simulink model "broadwayIPC_2024b"  (R2024b)
settings: Solver=FixedStepDiscrete  StartTime=0.0  StopTime=2  RelTol=1e-3
undefined symbols (not defined in the file or in its folder): gray
libraries: hdlsllib x26, visionhdlio x6, visionsources x2
Description:
  | Sobel Edge Detection Using the MATLAB(R) Function Block
  | This example shows how to use HDL Coder(TM) to check,
  | generate, and verify HDL code for a Sobel Edge Detection
  | block built using the MATLAB Function block.
settings Model: Creator=The MathWorks, Inc.  LastModifiedBy=Chris
settings SolverCC: AlgebraicLoopSolver=TrustRegion
settings DataIOCC: LimitDataPoints=on  SaveFormat=Array  SignalLogging=off  ReturnWorkspaceOutputs=off
settings OptimizationCC: BlockReduction=off  ConditionallyExecuteInputs=off  DefaultParameterBehavior=Inlined  ExpressionDepthLimit=2147483647  InitFltsAndDblsToZero=on  EfficientMapNaN2IntZero=off  LifeSpan=inf
settings DebuggingCC: AlgebraicLoopMsg=error  SaveWithParameterizedLinksMsg=none  UnderspecifiedInitializationDetection=Classic  MergeDetectMultiDrivingBlocksExec=none  SignalResolutionControl=TryResolveAllWithWarning  MultiTaskDSMMsg=warning  MultiTaskCondExecSysMsg=none  SingleTaskRateTransMsg=error  IntegerOverflowMsg=none  ParameterPrecisionLossMsg=none  FcnCallInpInsideContextMsg=warning  UnconnectedInputMsg=warning  UnconnectedOutputMsg=warning  UnconnectedLineMsg=warning  AllowSymbolicDim=off  StateNameClashWarn=warning  StrictBusMsg=ErrorOnBusTreatedAsVector  SFUnexpectedBacktrackingDiag=warning  SFNoUnconditionalDefaultTransitionDiag=warning  SFExecutionAtInitializationDiag=none  IntegerSaturationMsg=none  ArithmeticOperatorsInVariantConditions=warning
settings HardwareCC: ProdBitPerPointer=32  ProdBitPerSizeT=32  ProdBitPerPtrDiffT=32  ProdLargestAtomicFloat=None  ProdIntDivRoundTo=Undefined  ProdEndianess=Unspecified  ProdWordSize=32  ProdHWDeviceType=ASIC/FPGA  TargetHWDeviceType=32-bit Generic  ProdEqTarget=off
settings ModelReferenceCC: EnableRefExpFcnMdlSchedulingChecks=on  PropagateSignalLabelsOutOfModel=off
settings SFSimCC: SimUseLocalCustomCode=off  CustomCodeUndefinedFunction=UseInterfaceOnly
settings RTWCC: RTWUseLocalCustomCode=off  GPUComputeCapability=3.5  DLArmComputeVersion=19.05
settings CodeAppCC: StateflowObjectComments=on
settings GRTTargetCC: TargetFcnLib=ansi_tfl_tmw.mat  TargetLangStandard=C89/C90 (ANSI)  CombineOutputUpdateFcns=off  GRTInterface=on
settings ConfigComp: CovMetricSettings=dw  CovSaveCumulativeToWorkspaceVar=on  CovSaveSingleToWorkspaceVar=on  CovExternalEMLEnable=off

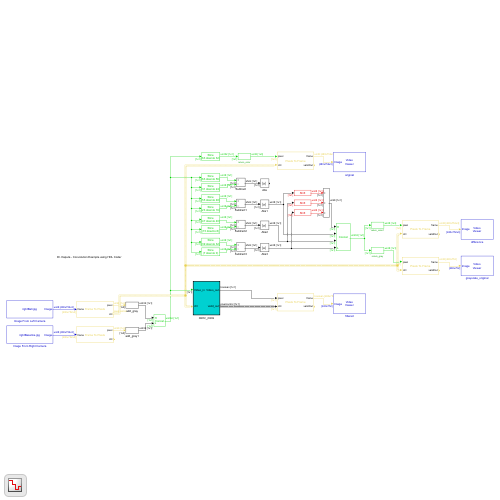
[thumbnail: Simulink's stored preview of the top-level diagram]
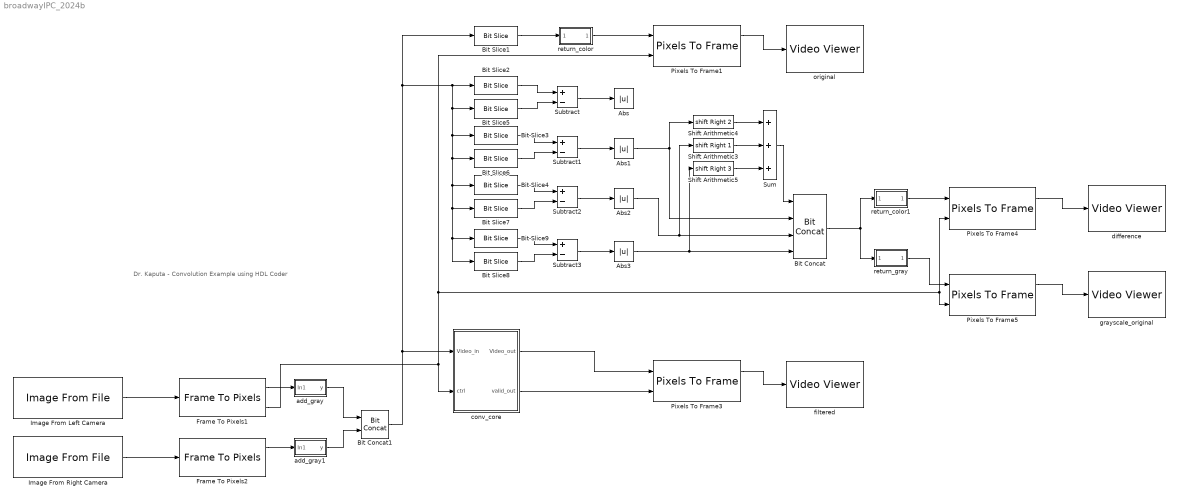
== system broadwayIPC_2024b ==
  note: Dr. Kaputa - Convolution Example using HDL Coder
  Abs{,1..3} (4 alike) : Abs  OutDataTypeStr=uint8
  Bit Concat : hdlsllib/Logic and Bit Operations/Bit Concat  numInputs=4
  Bit Concat1 : hdlsllib/Logic and Bit Operations/Bit Concat  numInputs=2
  Bit Slice1 : hdlsllib/Logic and Bit Operations/Bit Slice  lidx=63  ridx=32
  Bit Slice2 : hdlsllib/Logic and Bit Operations/Bit Slice  lidx=63  ridx=56
  Bit Slice3 : hdlsllib/Logic and Bit Operations/Bit Slice  lidx=55  ridx=48
  Bit Slice4 : hdlsllib/Logic and Bit Operations/Bit Slice  lidx=47  ridx=40
  Bit Slice5 : hdlsllib/Logic and Bit Operations/Bit Slice  lidx=31  ridx=24
  Bit Slice6 : hdlsllib/Logic and Bit Operations/Bit Slice  lidx=23  ridx=16
  Bit Slice7 : hdlsllib/Logic and Bit Operations/Bit Slice  lidx=15  ridx=8
  Bit Slice8 : hdlsllib/Logic and Bit Operations/Bit Slice  lidx=7  ridx=0
  Bit Slice9 : hdlsllib/Logic and Bit Operations/Bit Slice  lidx=39  ridx=32
  Frame To Pixels1 : visionhdlio/Frame To Pixels  NumComponents=3  NumPixels=1  VideoFormat=Custom  ActivePixelsPerLine=R  ActiveVideoLines=C  TotalPixelsPerLine=R  TotalVideoLines=C  StartingActiveLine=1  FrontPorch=0  SampleTime=0  VideoFormatCache=Custom  ActivePixelsPerLineCache=R  ActiveVideoLinesCache=C  TotalPixelsPerLineCache=R  TotalVideoLinesCache=C  StartingActiveLineCache=1  FrontPorchCache=0
  Frame To Pixels2 : visionhdlio/Frame To Pixels  NumComponents=3  NumPixels=1  VideoFormat=Custom  ActivePixelsPerLine=R  ActiveVideoLines=C  TotalPixelsPerLine=R  TotalVideoLines=C  StartingActiveLine=1  FrontPorch=0  SampleTime=0  VideoFormatCache=Custom  ActivePixelsPerLineCache=R  ActiveVideoLinesCache=C  TotalPixelsPerLineCache=R  TotalVideoLinesCache=C  StartingActiveLineCache=1  FrontPorchCache=0
  Image From Left Camera : visionsources/Image From File  Tag=vipblks_nd  FileName=C:\Users\Chris\Documents\Repos\WiiSports\TennisTracker\BoradwaySimulink\rightBall.jpg  Ts=1  imagePorts=One multidimensional signal  OutPortLabels=R|G|B  ImageDataType=Inherit from input image  sdImageDataType=uint(8)  Signed=on  WordLength=16  FractionLengthMode=User-defined  FractionLength=15
  Image From Right Camera : visionsources/Image From File  Tag=vipblks_nd  FileName=C:\Users\Chris\Documents\Repos\WiiSports\TennisTracker\BoradwaySimulink\rightBaseline.jpg  Ts=1  imagePorts=One multidimensional signal  OutPortLabels=R|G|B  ImageDataType=Inherit from input image  sdImageDataType=uint(8)  Signed=on  WordLength=16  FractionLengthMode=User-defined  FractionLength=15
  Pixels To Frame1 : visionhdlio/Pixels To Frame  NumComponents=3  NumPixels=1  VideoFormat=Custom  ActivePixelsPerLine=R  ActiveVideoLines=C  TotalPixelsPerLine=R  TotalVideoLines=C  VideoFormatCache=Custom  ActivePixelsPerLineCache=R  ActiveVideoLinesCache=C  TotalPixelsPerLineCache=R  TotalVideoLinesCache=C
  Pixels To Frame3 : visionhdlio/Pixels To Frame  NumComponents=1  NumPixels=1  VideoFormat=Custom  ActivePixelsPerLine=R  ActiveVideoLines=C  TotalPixelsPerLine=R  TotalVideoLines=C  VideoFormatCache=Custom  ActivePixelsPerLineCache=R  ActiveVideoLinesCache=C  TotalPixelsPerLineCache=R  TotalVideoLinesCache=C
  Pixels To Frame4 : visionhdlio/Pixels To Frame  NumComponents=3  NumPixels=1  VideoFormat=Custom  ActivePixelsPerLine=R  ActiveVideoLines=C  TotalPixelsPerLine=R  TotalVideoLines=C  VideoFormatCache=Custom  ActivePixelsPerLineCache=R  ActiveVideoLinesCache=C  TotalPixelsPerLineCache=R  TotalVideoLinesCache=C
  Pixels To Frame5 : visionhdlio/Pixels To Frame  NumComponents=1  NumPixels=1  VideoFormat=Custom  ActivePixelsPerLine=R  ActiveVideoLines=C  TotalPixelsPerLine=R  TotalVideoLines=C  VideoFormatCache=Custom  ActivePixelsPerLineCache=R  ActiveVideoLinesCache=C  TotalPixelsPerLineCache=R  TotalVideoLinesCache=C
  Shift Arithmetic3 : ArithShift  BitShiftNumber=1  BitShiftDirection=Right
  Shift Arithmetic4 : ArithShift  BitShiftNumber=2  BitShiftDirection=Right
  Shift Arithmetic5 : ArithShift  BitShiftNumber=3  BitShiftDirection=Right
  Subtract{,1..3} (4 alike) : Sum  Inputs=+-
  Sum : Sum  Inputs=+++  OutDataTypeStr=uint8
  add_gray : Subsystem
  add_gray1 : Subsystem
  conv_core : Subsystem  TreatAsAtomicUnit=on
  difference : VideoViewer  FigPos=[994 1078 927 429]
  filtered : VideoViewer  colormapValue=gray(256)  FigPos=[66 1078 927 429]
  grayscale_original : VideoViewer  FigPos=[65 538 927 429]
  original : VideoViewer  FigPos=[995 538 927 429]
  return_color : Subsystem
  return_color1 : Subsystem
  return_gray : Subsystem
  wires:
  Image From Left Camera/1 -> Frame To Pixels1/1
  Pixels To Frame1/1 -> original/1
  return_color/1(RGBVector) -> Pixels To Frame1/1
  Frame To Pixels1/1 -> add_gray/1(In1)
  Pixels To Frame3/1 -> filtered/1
  conv_core/2(valid_out) -> Pixels To Frame3/2
  Bit Concat1/1 -> Bit Slice1/1, Bit Slice2/1, Bit Slice8/1, Bit Slice9/1, Bit Slice7/1, Bit Slice4/1, Bit Slice6/1, Bit Slice3/1, Bit Slice5/1, conv_core/1(Video_in)
  conv_core/1(Video_out) -> Pixels To Frame3/1
  Image From Right Camera/1 -> Frame To Pixels2/1
  Frame To Pixels1/2 -> Pixels To Frame1/2, Pixels To Frame5/2, Pixels To Frame4/2, conv_core/2(ctrl)
  Frame To Pixels2/1 -> add_gray1/1(In1)
  add_gray/1(y) -> Bit Concat1/1
  add_gray1/1(y) -> Bit Concat1/2
  Bit Slice1/1 -> return_color/1(RGB)
  Pixels To Frame4/1 -> difference/1
  Subtract/1 -> Abs/1
  return_color1/1(RGBVector) -> Pixels To Frame4/1
  Subtract1/1 -> Abs1/1
  Subtract2/1 -> Abs2/1
  Subtract3/1 -> Abs3/1
  Bit Slice2/1 -> Subtract/1
  Bit Slice5/1 -> Subtract/2
  Bit Slice3/1 -> Subtract1/1
  Bit Slice6/1 -> Subtract1/2
  Bit Slice4/1 -> Subtract2/1
  Bit Slice7/1 -> Subtract2/2
  Bit Slice9/1 -> Subtract3/1
  Bit Slice8/1 -> Subtract3/2
  Pixels To Frame5/1 -> grayscale_original/1
  return_gray/1(RGBVector) -> Pixels To Frame5/1
  Shift Arithmetic5/1 -> Sum/3
  Shift Arithmetic3/1 -> Sum/2
  Shift Arithmetic4/1 -> Sum/1
  Abs3/1 -> Shift Arithmetic5/1, Bit Concat/4
  Abs2/1 -> Shift Arithmetic3/1, Bit Concat/3
  Abs1/1 -> Shift Arithmetic4/1, Bit Concat/2
  Sum/1 -> Bit Concat/1
  Bit Concat/1 -> return_gray/1(RGB), return_color1/1(RGB)

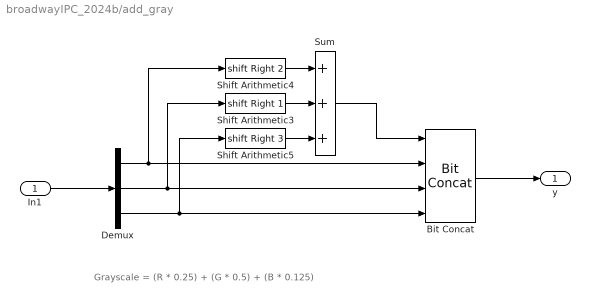
== system broadwayIPC_2024b/add_gray ==
  note: Grayscale = (R * 0.25) + (G * 0.5) + (B * 0.125)
  In1 : Inport
  Bit Concat : hdlsllib/Logic and Bit Operations/Bit Concat  numInputs=4
  Demux : Demux  Outputs=3
  Shift Arithmetic3 : ArithShift  BitShiftNumber=1  BitShiftDirection=Right
  Shift Arithmetic4 : ArithShift  BitShiftNumber=2  BitShiftDirection=Right
  Shift Arithmetic5 : ArithShift  BitShiftNumber=3  BitShiftDirection=Right
  Sum : Sum  Inputs=+++  OutDataTypeStr=uint8
  y : Outport
  wires:
  Bit Concat/1 -> y/1
  In1/1 -> Demux/1
  Demux/2 -> Shift Arithmetic3/1, Bit Concat/3
  Demux/1 -> Shift Arithmetic4/1, Bit Concat/2
  Demux/3 -> Shift Arithmetic5/1, Bit Concat/4
  Sum/1 -> Bit Concat/1
  Shift Arithmetic4/1 -> Sum/1
  Shift Arithmetic3/1 -> Sum/2
  Shift Arithmetic5/1 -> Sum/3

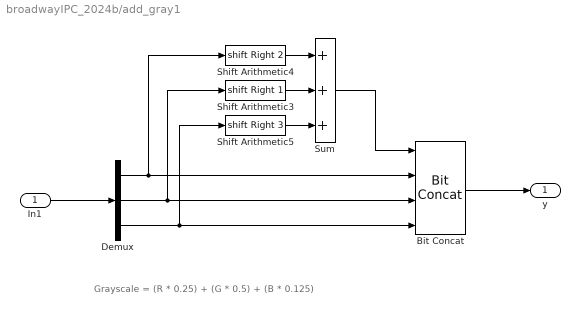
== system broadwayIPC_2024b/add_gray1 ==
  note: Grayscale = (R * 0.25) + (G * 0.5) + (B * 0.125)
  In1 : Inport
  Bit Concat : hdlsllib/Logic and Bit Operations/Bit Concat  numInputs=4
  Demux : Demux  Outputs=3
  Shift Arithmetic3 : ArithShift  BitShiftNumber=1  BitShiftDirection=Right
  Shift Arithmetic4 : ArithShift  BitShiftNumber=2  BitShiftDirection=Right
  Shift Arithmetic5 : ArithShift  BitShiftNumber=3  BitShiftDirection=Right
  Sum : Sum  Inputs=+++  OutDataTypeStr=uint8
  y : Outport
  wires:
  Bit Concat/1 -> y/1
  In1/1 -> Demux/1
  Demux/2 -> Shift Arithmetic3/1, Bit Concat/3
  Demux/1 -> Shift Arithmetic4/1, Bit Concat/2
  Demux/3 -> Shift Arithmetic5/1, Bit Concat/4
  Shift Arithmetic4/1 -> Sum/1
  Shift Arithmetic3/1 -> Sum/2
  Shift Arithmetic5/1 -> Sum/3
  Sum/1 -> Bit Concat/1

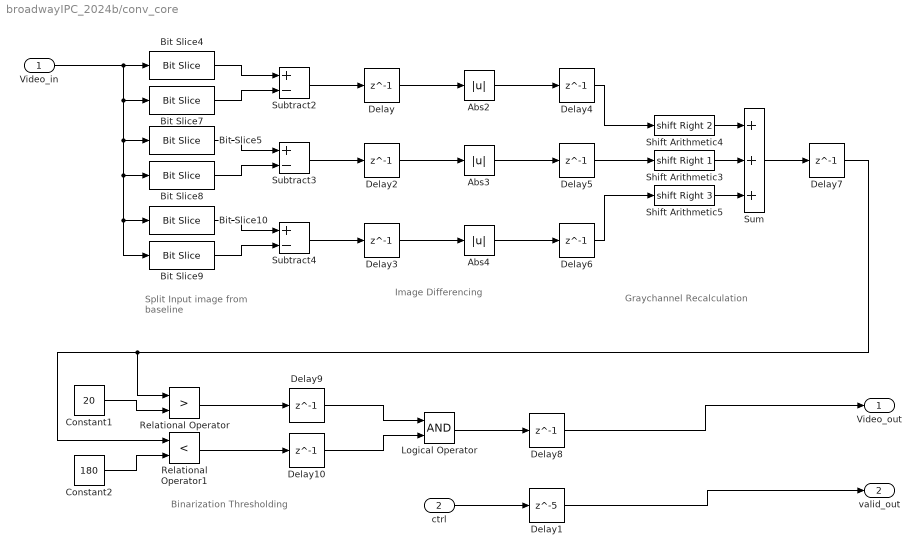
== system broadwayIPC_2024b/conv_core ==
  note: Graychannel Recalculation
  note: Split Input image
      | from baseline
  note: Image
      | Differencing
  note: Binarization Thresholding
  Video_in : Inport
  ctrl : Inport  Port=2
  Abs2 : Abs  OutDataTypeStr=uint8  SaturateOnIntegerOverflow=off
  Abs3 : Abs  OutDataTypeStr=uint8  SaturateOnIntegerOverflow=off
  Abs4 : Abs  OutDataTypeStr=uint8  SaturateOnIntegerOverflow=off
  Bit Slice10 : hdlsllib/Logic and Bit Operations/Bit Slice  lidx=39  ridx=32
  Bit Slice4 : hdlsllib/Logic and Bit Operations/Bit Slice  lidx=55  ridx=48
  Bit Slice5 : hdlsllib/Logic and Bit Operations/Bit Slice  lidx=47  ridx=40
  Bit Slice7 : hdlsllib/Logic and Bit Operations/Bit Slice  lidx=23  ridx=16
  Bit Slice8 : hdlsllib/Logic and Bit Operations/Bit Slice  lidx=15  ridx=8
  Bit Slice9 : hdlsllib/Logic and Bit Operations/Bit Slice  lidx=7  ridx=0
  Constant1 : Constant  Value=20  OutDataTypeStr=uint8
  Constant2 : Constant  Value=180  OutDataTypeStr=uint8
  Delay{,2..10} (10 alike) : Delay  DelayLength=1  InitialCondition=0
  Delay1 : Delay  DelayLength=5  InitialCondition=0
  Logical Operator : Logic  AllPortsSameDT=off  OutDataTypeStr=boolean
  Relational Operator : RelationalOperator  Operator=>  OutDataTypeStr=boolean  RndMeth=Simplest  InputSameDT=off
  Relational Operator1 : RelationalOperator  Operator=<  OutDataTypeStr=boolean  RndMeth=Simplest  InputSameDT=off
  Shift Arithmetic3 : ArithShift  BitShiftNumber=1  BitShiftDirection=Right
  Shift Arithmetic4 : ArithShift  BitShiftNumber=2  BitShiftDirection=Right
  Shift Arithmetic5 : ArithShift  BitShiftNumber=3  BitShiftDirection=Right
  Subtract2 : Sum  Inputs=+-
  Subtract3 : Sum  Inputs=+-
  Subtract4 : Sum  Inputs=+-
  Sum : Sum  Inputs=+++  OutDataTypeStr=uint8
  Video_out : Outport  VectorParamsAs1DForOutWhenUnconnected=off
  valid_out : Outport  Port=2  VectorParamsAs1DForOutWhenUnconnected=off
  wires:
  ctrl/1 -> Delay1/1
  Constant1/1 -> Relational Operator/2
  Constant2/1 -> Relational Operator1/2
  Abs2/1 -> Delay4/1
  Bit Slice9/1 -> Subtract4/2
  Bit Slice7/1 -> Subtract2/2
  Bit Slice4/1 -> Subtract2/1
  Bit Slice10/1 -> Subtract4/1
  Abs3/1 -> Delay5/1
  Bit Slice5/1 -> Subtract3/1
  Bit Slice8/1 -> Subtract3/2
  Abs4/1 -> Delay6/1
  Video_in/1 -> Bit Slice9/1, Bit Slice10/1, Bit Slice8/1, Bit Slice5/1, Bit Slice7/1, Bit Slice4/1
  Sum/1 -> Delay7/1
  Shift Arithmetic4/1 -> Sum/1
  Shift Arithmetic5/1 -> Sum/3
  Shift Arithmetic3/1 -> Sum/2
  Subtract2/1 -> Delay/1
  Delay/1 -> Abs2/1
  Subtract3/1 -> Delay2/1
  Delay2/1 -> Abs3/1
  Subtract4/1 -> Delay3/1
  Delay3/1 -> Abs4/1
  Delay4/1 -> Shift Arithmetic4/1
  Delay5/1 -> Shift Arithmetic3/1
  Delay6/1 -> Shift Arithmetic5/1
  Delay7/1 -> Relational Operator/1, Relational Operator1/1
  Logical Operator/1 -> Delay8/1
  Relational Operator/1 -> Delay9/1
  Relational Operator1/1 -> Delay10/1
  Delay10/1 -> Logical Operator/2
  Delay9/1 -> Logical Operator/1
  Delay8/1 -> Video_out/1
  Delay1/1 -> valid_out/1

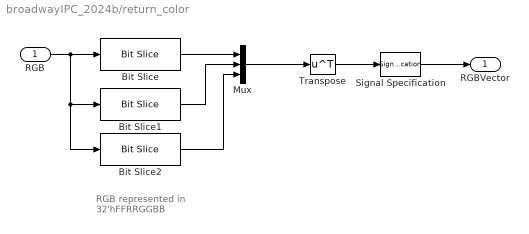
== system broadwayIPC_2024b/return_color ==
  note: RGB represented in
      | 32'hFFRRGGBB
  RGB : Inport
  Bit Slice : hdlsllib/Logic and Bit Operations/Bit Slice  lidx=23  ridx=16
  Bit Slice1 : hdlsllib/Logic and Bit Operations/Bit Slice  lidx=15  ridx=8
  Bit Slice2 : hdlsllib/Logic and Bit Operations/Bit Slice  lidx=7  ridx=0
  Mux : Mux  Inputs=3
  Signal Specification : SignalSpecification
  Transpose : Math  Operator=transpose  SignedPower=on
  RGBVector : Outport  VectorParamsAs1DForOutWhenUnconnected=off
  wires:
  Signal Specification/1 -> RGBVector/1
  Transpose/1 -> Signal Specification/1
  RGB/1 -> Bit Slice/1, Bit Slice1/1, Bit Slice2/1
  Bit Slice1/1 -> Mux/2
  Bit Slice2/1 -> Mux/3
  Bit Slice/1 -> Mux/1
  Mux/1 -> Transpose/1

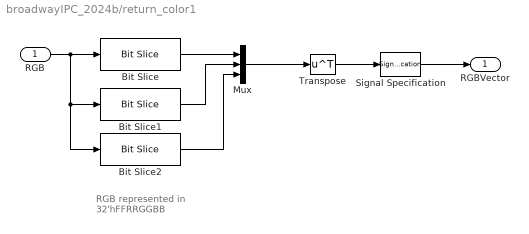
== system broadwayIPC_2024b/return_color1 ==
  note: RGB represented in
      | 32'hFFRRGGBB
  RGB : Inport
  Bit Slice : hdlsllib/Logic and Bit Operations/Bit Slice  lidx=23  ridx=16
  Bit Slice1 : hdlsllib/Logic and Bit Operations/Bit Slice  lidx=15  ridx=8
  Bit Slice2 : hdlsllib/Logic and Bit Operations/Bit Slice  lidx=7  ridx=0
  Mux : Mux  Inputs=3
  Signal Specification : SignalSpecification
  Transpose : Math  Operator=transpose  SignedPower=on
  RGBVector : Outport  VectorParamsAs1DForOutWhenUnconnected=off
  wires:
  Signal Specification/1 -> RGBVector/1
  Transpose/1 -> Signal Specification/1
  RGB/1 -> Bit Slice/1, Bit Slice1/1, Bit Slice2/1
  Bit Slice1/1 -> Mux/2
  Bit Slice2/1 -> Mux/3
  Bit Slice/1 -> Mux/1
  Mux/1 -> Transpose/1

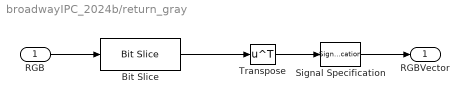
== system broadwayIPC_2024b/return_gray ==
  RGB : Inport
  Bit Slice : hdlsllib/Logic and Bit Operations/Bit Slice  lidx=31  ridx=24
  Signal Specification : SignalSpecification
  Transpose : Math  Operator=transpose  SignedPower=on
  RGBVector : Outport  VectorParamsAs1DForOutWhenUnconnected=off
  wires:
  RGB/1 -> Bit Slice/1
  Transpose/1 -> Signal Specification/1
  Signal Specification/1 -> RGBVector/1
  Bit Slice/1 -> Transpose/1
